simulink model "npc_angle"  (R2019b)
settings: Solver=FixedStepDiscrete  StartTime=0.0  StopTime=0.5  FixedStep=Ts  RelTol=1e-3
values from neighbouring files (symbols this model uses):
  Ts = 1.0/50000.0    (= 2e-05)    [m_npc_angle.m]
undefined symbols (not defined in the file or in its folder): DiscIntNeverNeededParam
settings Model: Creator=Dmitry  LastModifiedBy=NPT

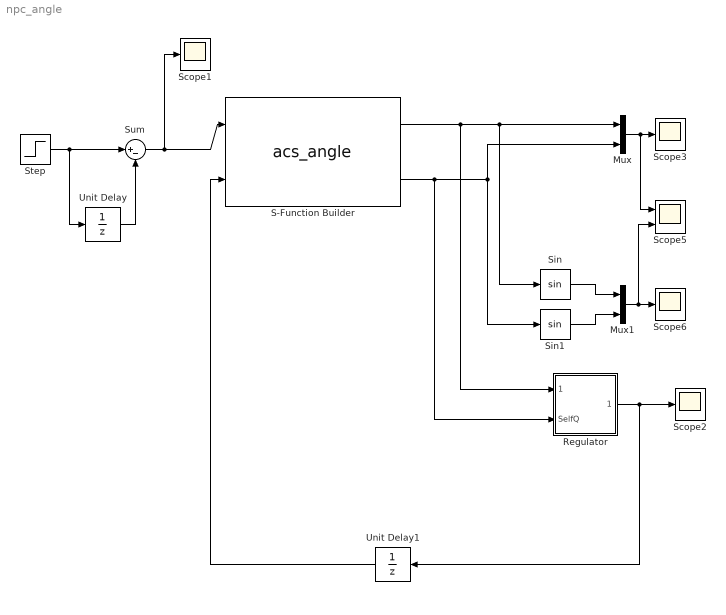
== system npc_angle ==
  Mux : Mux  Inputs=2
  Mux1 : Mux  Inputs=2
  Regulator : Subsystem
  S-Function Builder : S-Function  InitFcn=try, set_param(gcb,'FunctionName','acs_angle'), end  FunctionName=acs_angle  Parameters=Ts  SFunctionModules=acs_angle_wrapper itrans_func integrator  SFunctionDeploymentMode=off  EnableBusSupport=off  mask(S-Function Builder){}
      mask help: Simulink:masks:SFunctionBuilder_MD
      mask init:
      | val = [[.9  0.75 0.75 1 1 .9 .9 1]',[1 1 0.75 0.75 .9 .9 1 .9]'];try , sys = get_param(gcb,'SfunBuilderFcnName');if isempty(sys), sys = get_param(gcb,'FunctionName'); end,catch, sys = get_param(gcb,'FunctionName'); end
      settings: CopyFcn=set_param(gcbh,'LinkStatus','none')  PreSaveFcn=try, set_param(gcb,'FunctionName','acs_angle'), end  OpenFcn=sfunctionwizard(gcbh)
      mask Display: plot(val(:,1),val(:,2)),disp(sys), port_label('input',1,'rand'), port_label('input',2,'errQ'), port_label('output',1,'RemoteQ'), port_label('output',2,'SelfQ')
  Scope{1..3,6} (4 alike) : Scope
  Scope5 : Scope  NumInputPorts=2
  Sin : Trigonometry
  Sin1 : Trigonometry
  Step : Step  Time=0.005  After=0.52  SampleTime=Ts
  Sum : Sum  Inputs=|+-
  Unit Delay : UnitDelay  SampleTime=Ts  HasFrameUpgradeWarning=on
  Unit Delay1 : UnitDelay  SampleTime=Ts  HasFrameUpgradeWarning=on
  wires:
  S-Function Builder/1 -> Regulator/1(RemoteQ), Sin/1, Mux/1
  Step/1 -> Unit Delay/1, Sum/1
  Sum/1 -> S-Function Builder/1, Scope1/1
  Unit Delay/1 -> Sum/2
  S-Function Builder/2 -> Regulator/2(SelfQ), Sin1/1, Mux/2
  Mux/1 -> Scope5/1, Scope3/1
  Mux1/1 -> Scope5/2, Scope6/1
  Unit Delay1/1 -> S-Function Builder/2
  Regulator/1(deltaQ) -> Scope2/1, Unit Delay1/1
  Sin/1 -> Mux1/1
  Sin1/1 -> Mux1/2

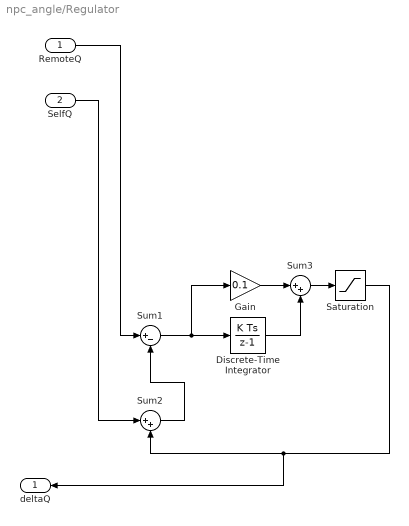
== system npc_angle/Regulator ==
  RemoteQ : Inport
  SelfQ : Inport  Port=2
  Discrete-Time Integrator : DiscreteIntegrator  gainval=0.0001  SampleTime=Ts  LimitOutput=on  UpperSaturationLimit=pi  LowerSaturationLimit=-pi  ICPrevOutput=DiscIntNeverNeededParam  ICPrevScaledInput=DiscIntNeverNeededParam
  Gain : Gain  Gain=0.1
  Saturation : Saturate  UpperLimit=pi  LowerLimit=-pi
  Sum1 : Sum  Inputs=|+-
  Sum2 : Sum  Inputs=|++
  Sum3 : Sum  Inputs=|++
  deltaQ : Outport
  wires:
  Saturation/1 -> deltaQ/1, Sum2/2
  Sum3/1 -> Saturation/1
  Sum1/1 -> Gain/1, Discrete-Time Integrator/1
  Sum2/1 -> Sum1/2
  Discrete-Time Integrator/1 -> Sum3/2
  RemoteQ/1 -> Sum1/1
  SelfQ/1 -> Sum2/1
  Gain/1 -> Sum3/1
